simulink model "simulation_workspace"  (R2020b)
settings: Solver=VariableStepAuto  StartTime=0.0  StopTime=10.0  RelTol=1e-3
undefined symbols (not defined in the file or in its folder): Ac, Bc, Cc, Dc
settings Model: Creator=jvalencia  LastModifiedBy=jvalencia

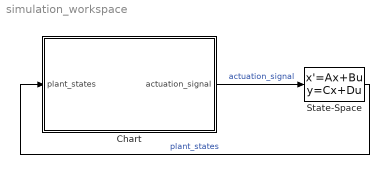
== system simulation_workspace ==
  Chart : Stateflow chart  TreatAsAtomicUnit=on
  State-Space : StateSpace  A=Ac  B=Bc  C=Cc  D=Dc  InitialCondition=0  ContinuousStateAttributes={'s0','s1','s2'}
  wires:
  Chart/1(actuation_signal) -> State-Space/1  "actuation_signal"
  State-Space/1 -> Chart/1(plant_states)  "plant_states"

== stateflow chart simulation_workspace/Chart ==
  state modeSwitching
    state ?
    state start
      en:
      i = 0;
      du: i = i + 1;
    (default) -> (junction 14)
    (junction 14) -> start : [mode == 1]
  data: switching_sequence function_input; sampling_intervals function_input; sampling_interval function_output; actuation_signal output; plant_states input
  function sampling_interval  = getSamplingInterval(switching_sequence, sampling_intervals):
    | function sampling_interval  = getSamplingInterval(switching_sequence, sampling_intervals)
    | 
    | sampling_interval = sampling_intervals(switching_sequence);
    | 
    | end
